simulink model "Template_v4_00_2023a_Jetson"  (R2023a)
settings: Solver=ode4  StartTime=0.0  StopTime=tsim  FixedStep=baseRate  RelTol=1e-6  AbsTol=1e-6
values from neighbouring files (symbols this model uses):
  a1 = shape(1)    [Cardioid.m]    (also in Run_Initializer.m = 0.3)
  a2 = shape(2)    [Cardioid.m]    (also in Run_Initializer.m = 0.3)
  a3 = shape(3)    [Cardioid.m]    (also in Run_Initializer.m = 0.4)
  b1 = shape(4)    [Cardioid.m]    (also in Run_Initializer.m = 0.175)
  b2 = shape(5)    [Cardioid.m]    (also in Run_Initializer.m = 0.175)
  drop_states_BLACK = BLACK_ini(1:3)    [Run_Initializer.m]
  drop_states_BLUE = BLUE_ini(1:3)    [Run_Initializer.m]
  drop_states_RED = RED_ini(1:3)    [Run_Initializer.m]
  Gamma1_el = 0.12    [Run_Initializer.m]
  Gamma1_sh = 0.005    [Run_Initializer.m]
  Gamma1_wr = 0.025    [Run_Initializer.m]
  Gamma2_el = 5    [Run_Initializer.m]
  Gamma2_sh = 5    [Run_Initializer.m]
  Gamma2_wr = 5    [Run_Initializer.m]
  Gamma3_el = 10    [Run_Initializer.m]
  Gamma3_sh = 40    [Run_Initializer.m]
  Gamma3_wr = 40    [Run_Initializer.m]
  Gamma4_el = 0.039    [Run_Initializer.m]
  Gamma4_sh = 0.015    [Run_Initializer.m]
  Gamma4_wr = 0.029    [Run_Initializer.m]
  Gamma5_el = 800    [Run_Initializer.m]
  Gamma5_sh = 800    [Run_Initializer.m]
  Gamma5_wr = 800    [Run_Initializer.m]
  Gamma6_el = 0.000001    (= 1e-06)    [Run_Initializer.m]
  Gamma6_sh = 0.005    [Run_Initializer.m]
  Gamma6_wr = 0.02    [Run_Initializer.m]
  home_states_BLACK = BLACK_ini(1:3)    [Run_Initializer.m]
  home_states_BLUE = BLUE_ini(1:3)    [Run_Initializer.m]
  home_states_RED = RED_ini(1:3)    [Run_Initializer.m]
  init_states_BLACK = BLACK_ini(1:3)    [Run_Initializer.m]
  init_states_BLUE = BLUE_ini(1:3)    [Run_Initializer.m]
  init_states_RED = RED_ini(1:3)    [Run_Initializer.m]
  Kd_elarm = 0.8    [Run_Initializer.m]
  Kd_sharm = 1.0    (= 1)    [Run_Initializer.m]
  Kd_wrarm = 0.6    [Run_Initializer.m]
  Kp_elarm = 1.2    [Run_Initializer.m]
  Kp_sharm = 1.5    [Run_Initializer.m]
  Kp_wrarm = 2    [Run_Initializer.m]
  PWMFreq = 5    [Run_Initializer.m]
  Tz_lim_elarm = .1    (= 0.1)    [Run_Initializer.m]
  Tz_lim_sharm = .1    (= 0.1)    [Run_Initializer.m]
  Tz_lim_wrarm = .1    (= 0.1)    [Run_Initializer.m]
undefined symbols (not defined in the file or in its folder): b0, b3, baseRate, DiscIntNeverNeededParam, drop_states_ARM, F_Black_X_nominal, F_Black_Y_nominal, F_Blue_X_nominal, F_Blue_Y_nominal, F_red_X_nominal, F_red_Y_nominal, F_thrusters_BLACK, F_thrusters_BLUE, F_thrusters_RED, IBLACK, IBLUE, IDIST, IEE, IPROX, IRED, Kd_tb, Kd_tblue, Kd_tr, Kd_xb, Kd_xblue, Kd_xr, Kd_yb, Kd_yblue, Kd_yr, Kp_tb, Kp_tblue, Kp_tr, Kp_xb, Kp_xblue, Kp_xr, Kp_yb, Kp_yblue, Kp_yr, mBLACK, mBLUE, mDIST, mEE, mPROX, mRED, noise_variance_BLACK, noise_variance_BLUE, noise_variance_RED, Phase0_End, Phase1_End, Phase2_End, Phase3_End, Phase3_SubPhase1_End, Phase3_SubPhase2_End, Phase3_SubPhase3_End, Phase3_SubPhase4_End, Phase4_End, Phase5_End, Phi, platformSelection, serverRate ... (+6)
libraries: nvidiaSharedBlocks x9, MainLibrary x4, dspsigops x4, simulink x1
(part 8 of 11)

== system Template_v4_00_2023a_Jetson/Phase #3: Experiment/Change BLACK Behavior/Sub-Phase #4/BLACK_RzD/Wrap1 ==
  unwrapped : Inport
  MATLAB Function : MATLAB Function  TreatAsAtomicUnit=on
  wrapped : Outport  VectorParamsAs1DForOutWhenUnconnected=off
  wires:
  MATLAB Function/1(wrappedAngle) -> wrapped/1
  unwrapped/1 -> MATLAB Function/1(u)

== system Template_v4_00_2023a_Jetson/Phase #3: Experiment/Change BLACK Behavior/Sub-Phase #4/Custom Discrete PD (Attitude)/x_dot -> x1 ==
  note: dy/dt ~= (y2-y1)/deltaT
  y(t) : Inport
  Delay1 : Delay  DelayLength=1  InitialConditionSource=Input port
      settings: InputPortMap=u0,p4
  Hold this value : Subsystem  TreatAsAtomicUnit=on
  Sum6 : Sum  Inputs=-+|
  divide by delta T : Gain  Gain=1/baseRate
  "if we went through a \"step\"" : If  IfExpression=u1 ~= 0  ShowElse=off
  dy(t)/dt : Outport  VectorParamsAs1DForOutWhenUnconnected=off
  wires:
  divide by delta T/1 -> dy(t)/dt/1
  Delay1/1 -> Sum6/1
  "if we went through a \"step\""/1 -> Hold this value/Action
  Hold this value/1(Out1) -> divide by delta T/1
  Sum6/1 -> "if we went through a \"step\""/1, Hold this value/1(In1)
  y(t)/1 -> Sum6/2, Delay1/2, Delay1/1

== system Template_v4_00_2023a_Jetson/Phase #3: Experiment/Change BLACK Behavior/Sub-Phase #4/Custom Discrete PD (X-Position)/x_dot -> x1 ==
  note: dy/dt ~= (y2-y1)/deltaT
  y(t) : Inport
  Delay1 : Delay  DelayLength=1  InitialConditionSource=Input port
      settings: InputPortMap=u0,p4
  Hold this value : Subsystem  TreatAsAtomicUnit=on
  Sum6 : Sum  Inputs=-+|
  divide by delta T : Gain  Gain=1/baseRate
  "if we went through a \"step\"" : If  IfExpression=u1 ~= 0  ShowElse=off
  dy(t)/dt : Outport  VectorParamsAs1DForOutWhenUnconnected=off
  wires:
  divide by delta T/1 -> dy(t)/dt/1
  Delay1/1 -> Sum6/1
  "if we went through a \"step\""/1 -> Hold this value/Action
  Hold this value/1(Out1) -> divide by delta T/1
  Sum6/1 -> "if we went through a \"step\""/1, Hold this value/1(In1)
  y(t)/1 -> Sum6/2, Delay1/2, Delay1/1

== system Template_v4_00_2023a_Jetson/Phase #3: Experiment/Change BLACK Behavior/Sub-Phase #4/Custom Discrete PD (Y-Position)/x_dot -> x1 ==
  note: dy/dt ~= (y2-y1)/deltaT
  y(t) : Inport
  Delay1 : Delay  DelayLength=1  InitialConditionSource=Input port
      settings: InputPortMap=u0,p4
  Hold this value : Subsystem  TreatAsAtomicUnit=on
  Sum6 : Sum  Inputs=-+|
  divide by delta T : Gain  Gain=1/baseRate
  "if we went through a \"step\"" : If  IfExpression=u1 ~= 0  ShowElse=off
  dy(t)/dt : Outport  VectorParamsAs1DForOutWhenUnconnected=off
  wires:
  divide by delta T/1 -> dy(t)/dt/1
  Delay1/1 -> Sum6/1
  "if we went through a \"step\""/1 -> Hold this value/Action
  Hold this value/1(Out1) -> divide by delta T/1
  Sum6/1 -> "if we went through a \"step\""/1, Hold this value/1(In1)
  y(t)/1 -> Sum6/2, Delay1/2, Delay1/1

== system Template_v4_00_2023a_Jetson/Phase #3: Experiment/Change BLUE Behavior/Sub-Phase #1/BLUE_Rz Desired/Subsystem ==
  Constant1 : Constant  Value=Phase2_End  SampleTime=-1
  Subtract : Sum  Inputs=+-
  Universal_Time : DataStoreRead  DataStoreName=Univ_Time  IndexOptions=Index vector (dialog)  Indices=1  OutputSizes=1
  Time : Outport  VectorParamsAs1DForOutWhenUnconnected=off
  wires:
  Universal_Time/1 -> Subtract/1
  Subtract/1 -> Time/1
  Constant1/1 -> Subtract/2

== system Template_v4_00_2023a_Jetson/Phase #3: Experiment/Change BLUE Behavior/Sub-Phase #1/BLUE_Rz Desired/Wrap ==
  unwrapped : Inport
  MATLAB Function : MATLAB Function  TreatAsAtomicUnit=on
  wrapped : Outport  VectorParamsAs1DForOutWhenUnconnected=off
  wires:
  MATLAB Function/1(wrappedAngle) -> wrapped/1
  unwrapped/1 -> MATLAB Function/1(u)

== system Template_v4_00_2023a_Jetson/Phase #3: Experiment/Change BLUE Behavior/Sub-Phase #1/Custom Discrete PD (Attitude)/x_dot -> x1 ==
  note: dy/dt ~= (y2-y1)/deltaT
  y(t) : Inport
  Delay1 : Delay  DelayLength=1  InitialConditionSource=Input port
      settings: InputPortMap=u0,p4
  Hold this value : Subsystem  TreatAsAtomicUnit=on
  Sum6 : Sum  Inputs=-+|
  divide by delta T : Gain  Gain=1/baseRate
  "if we went through a \"step\"" : If  IfExpression=u1 ~= 0  ShowElse=off
  dy(t)/dt : Outport  VectorParamsAs1DForOutWhenUnconnected=off
  wires:
  divide by delta T/1 -> dy(t)/dt/1
  Delay1/1 -> Sum6/1
  "if we went through a \"step\""/1 -> Hold this value/Action
  Hold this value/1(Out1) -> divide by delta T/1
  Sum6/1 -> "if we went through a \"step\""/1, Hold this value/1(In1)
  y(t)/1 -> Sum6/2, Delay1/2, Delay1/1

== system Template_v4_00_2023a_Jetson/Phase #3: Experiment/Change BLUE Behavior/Sub-Phase #1/Custom Discrete PD (X-Position)/x_dot -> x1 ==
  note: dy/dt ~= (y2-y1)/deltaT
  y(t) : Inport
  Delay1 : Delay  DelayLength=1  InitialConditionSource=Input port
      settings: InputPortMap=u0,p4
  Hold this value : Subsystem  TreatAsAtomicUnit=on
  Sum6 : Sum  Inputs=-+|
  divide by delta T : Gain  Gain=1/baseRate
  "if we went through a \"step\"" : If  IfExpression=u1 ~= 0  ShowElse=off
  dy(t)/dt : Outport  VectorParamsAs1DForOutWhenUnconnected=off
  wires:
  divide by delta T/1 -> dy(t)/dt/1
  Delay1/1 -> Sum6/1
  "if we went through a \"step\""/1 -> Hold this value/Action
  Hold this value/1(Out1) -> divide by delta T/1
  Sum6/1 -> "if we went through a \"step\""/1, Hold this value/1(In1)
  y(t)/1 -> Sum6/2, Delay1/2, Delay1/1

== system Template_v4_00_2023a_Jetson/Phase #3: Experiment/Change BLUE Behavior/Sub-Phase #1/Custom Discrete PD (Y-Position)/x_dot -> x1 ==
  note: dy/dt ~= (y2-y1)/deltaT
  y(t) : Inport
  Delay1 : Delay  DelayLength=1  InitialConditionSource=Input port
      settings: InputPortMap=u0,p4
  Hold this value : Subsystem  TreatAsAtomicUnit=on
  Sum6 : Sum  Inputs=-+|
  divide by delta T : Gain  Gain=1/baseRate
  "if we went through a \"step\"" : If  IfExpression=u1 ~= 0  ShowElse=off
  dy(t)/dt : Outport  VectorParamsAs1DForOutWhenUnconnected=off
  wires:
  divide by delta T/1 -> dy(t)/dt/1
  Delay1/1 -> Sum6/1
  "if we went through a \"step\""/1 -> Hold this value/Action
  Hold this value/1(Out1) -> divide by delta T/1
  Sum6/1 -> "if we went through a \"step\""/1, Hold this value/1(In1)
  y(t)/1 -> Sum6/2, Delay1/2, Delay1/1

== system Template_v4_00_2023a_Jetson/Phase #3: Experiment/Change BLUE Behavior/Sub-Phase #1/Subsystem2/Subsystem ==
  Universal_Time : DataStoreRead  DataStoreName=Univ_Time  IndexOptions=Index vector (dialog)  Indices=1  OutputSizes=1
  Time : Outport  VectorParamsAs1DForOutWhenUnconnected=off
  wires:
  Universal_Time/1 -> Time/1

== system Template_v4_00_2023a_Jetson/Phase #3: Experiment/Change BLUE Behavior/Sub-Phase #2 /BLUE_Rz Desired/Subsystem ==
  Constant1 : Constant  Value=Phase2_End  SampleTime=-1
  Subtract : Sum  Inputs=+-
  Universal_Time : DataStoreRead  DataStoreName=Univ_Time  IndexOptions=Index vector (dialog)  Indices=1  OutputSizes=1
  Time : Outport  VectorParamsAs1DForOutWhenUnconnected=off
  wires:
  Universal_Time/1 -> Subtract/1
  Subtract/1 -> Time/1
  Constant1/1 -> Subtract/2

== system Template_v4_00_2023a_Jetson/Phase #3: Experiment/Change BLUE Behavior/Sub-Phase #2 /BLUE_Rz Desired/Wrap ==
  unwrapped : Inport
  MATLAB Function : MATLAB Function  TreatAsAtomicUnit=on
  wrapped : Outport  VectorParamsAs1DForOutWhenUnconnected=off
  wires:
  MATLAB Function/1(wrappedAngle) -> wrapped/1
  unwrapped/1 -> MATLAB Function/1(u)

== system Template_v4_00_2023a_Jetson/Phase #3: Experiment/Change BLUE Behavior/Sub-Phase #2 /Custom Discrete PD (Attitude)/x_dot -> x1 ==
  note: dy/dt ~= (y2-y1)/deltaT
  y(t) : Inport
  Delay1 : Delay  DelayLength=1  InitialConditionSource=Input port
      settings: InputPortMap=u0,p4
  Hold this value : Subsystem  TreatAsAtomicUnit=on
  Sum6 : Sum  Inputs=-+|
  divide by delta T : Gain  Gain=1/baseRate
  "if we went through a \"step\"" : If  IfExpression=u1 ~= 0  ShowElse=off
  dy(t)/dt : Outport  VectorParamsAs1DForOutWhenUnconnected=off
  wires:
  divide by delta T/1 -> dy(t)/dt/1
  Delay1/1 -> Sum6/1
  "if we went through a \"step\""/1 -> Hold this value/Action
  Hold this value/1(Out1) -> divide by delta T/1
  Sum6/1 -> "if we went through a \"step\""/1, Hold this value/1(In1)
  y(t)/1 -> Sum6/2, Delay1/2, Delay1/1

== system Template_v4_00_2023a_Jetson/Phase #3: Experiment/Change BLUE Behavior/Sub-Phase #2 /Custom Discrete PD (X-Position)/x_dot -> x1 ==
  note: dy/dt ~= (y2-y1)/deltaT
  y(t) : Inport
  Delay1 : Delay  DelayLength=1  InitialConditionSource=Input port
      settings: InputPortMap=u0,p4
  Hold this value : Subsystem  TreatAsAtomicUnit=on
  Sum6 : Sum  Inputs=-+|
  divide by delta T : Gain  Gain=1/baseRate
  "if we went through a \"step\"" : If  IfExpression=u1 ~= 0  ShowElse=off
  dy(t)/dt : Outport  VectorParamsAs1DForOutWhenUnconnected=off
  wires:
  divide by delta T/1 -> dy(t)/dt/1
  Delay1/1 -> Sum6/1
  "if we went through a \"step\""/1 -> Hold this value/Action
  Hold this value/1(Out1) -> divide by delta T/1
  Sum6/1 -> "if we went through a \"step\""/1, Hold this value/1(In1)
  y(t)/1 -> Sum6/2, Delay1/2, Delay1/1

== system Template_v4_00_2023a_Jetson/Phase #3: Experiment/Change BLUE Behavior/Sub-Phase #2 /Custom Discrete PD (Y-Position)/x_dot -> x1 ==
  note: dy/dt ~= (y2-y1)/deltaT
  y(t) : Inport
  Delay1 : Delay  DelayLength=1  InitialConditionSource=Input port
      settings: InputPortMap=u0,p4
  Hold this value : Subsystem  TreatAsAtomicUnit=on
  Sum6 : Sum  Inputs=-+|
  divide by delta T : Gain  Gain=1/baseRate
  "if we went through a \"step\"" : If  IfExpression=u1 ~= 0  ShowElse=off
  dy(t)/dt : Outport  VectorParamsAs1DForOutWhenUnconnected=off
  wires:
  divide by delta T/1 -> dy(t)/dt/1
  Delay1/1 -> Sum6/1
  "if we went through a \"step\""/1 -> Hold this value/Action
  Hold this value/1(Out1) -> divide by delta T/1
  Sum6/1 -> "if we went through a \"step\""/1, Hold this value/1(In1)
  y(t)/1 -> Sum6/2, Delay1/2, Delay1/1

== system Template_v4_00_2023a_Jetson/Phase #3: Experiment/Change BLUE Behavior/Sub-Phase #2 /Subsystem2/Subsystem ==
  Universal_Time : DataStoreRead  DataStoreName=Univ_Time  IndexOptions=Index vector (dialog)  Indices=1  OutputSizes=1
  Time : Outport  VectorParamsAs1DForOutWhenUnconnected=off
  wires:
  Universal_Time/1 -> Time/1

== system Template_v4_00_2023a_Jetson/Phase #3: Experiment/Change BLUE Behavior/Sub-Phase #3 /BLUE_Rz Desired/Subsystem ==
  Constant1 : Constant  Value=Phase2_End  SampleTime=-1
  Subtract : Sum  Inputs=+-
  Universal_Time : DataStoreRead  DataStoreName=Univ_Time  IndexOptions=Index vector (dialog)  Indices=1  OutputSizes=1
  Time : Outport  VectorParamsAs1DForOutWhenUnconnected=off
  wires:
  Universal_Time/1 -> Subtract/1
  Subtract/1 -> Time/1
  Constant1/1 -> Subtract/2

== system Template_v4_00_2023a_Jetson/Phase #3: Experiment/Change BLUE Behavior/Sub-Phase #3 /BLUE_Rz Desired/Wrap ==
  unwrapped : Inport
  MATLAB Function : MATLAB Function  TreatAsAtomicUnit=on
  wrapped : Outport  VectorParamsAs1DForOutWhenUnconnected=off
  wires:
  MATLAB Function/1(wrappedAngle) -> wrapped/1
  unwrapped/1 -> MATLAB Function/1(u)

== system Template_v4_00_2023a_Jetson/Phase #3: Experiment/Change BLUE Behavior/Sub-Phase #3 /Custom Discrete PD (Attitude)/x_dot -> x1 ==
  note: dy/dt ~= (y2-y1)/deltaT
  y(t) : Inport
  Delay1 : Delay  DelayLength=1  InitialConditionSource=Input port
      settings: InputPortMap=u0,p4
  Hold this value : Subsystem  TreatAsAtomicUnit=on
  Sum6 : Sum  Inputs=-+|
  divide by delta T : Gain  Gain=1/baseRate
  "if we went through a \"step\"" : If  IfExpression=u1 ~= 0  ShowElse=off
  dy(t)/dt : Outport  VectorParamsAs1DForOutWhenUnconnected=off
  wires:
  divide by delta T/1 -> dy(t)/dt/1
  Delay1/1 -> Sum6/1
  "if we went through a \"step\""/1 -> Hold this value/Action
  Hold this value/1(Out1) -> divide by delta T/1
  Sum6/1 -> "if we went through a \"step\""/1, Hold this value/1(In1)
  y(t)/1 -> Sum6/2, Delay1/2, Delay1/1

== system Template_v4_00_2023a_Jetson/Phase #3: Experiment/Change BLUE Behavior/Sub-Phase #3 /Custom Discrete PD (X-Position)/x_dot -> x1 ==
  note: dy/dt ~= (y2-y1)/deltaT
  y(t) : Inport
  Delay1 : Delay  DelayLength=1  InitialConditionSource=Input port
      settings: InputPortMap=u0,p4
  Hold this value : Subsystem  TreatAsAtomicUnit=on
  Sum6 : Sum  Inputs=-+|
  divide by delta T : Gain  Gain=1/baseRate
  "if we went through a \"step\"" : If  IfExpression=u1 ~= 0  ShowElse=off
  dy(t)/dt : Outport  VectorParamsAs1DForOutWhenUnconnected=off
  wires:
  divide by delta T/1 -> dy(t)/dt/1
  Delay1/1 -> Sum6/1
  "if we went through a \"step\""/1 -> Hold this value/Action
  Hold this value/1(Out1) -> divide by delta T/1
  Sum6/1 -> "if we went through a \"step\""/1, Hold this value/1(In1)
  y(t)/1 -> Sum6/2, Delay1/2, Delay1/1

== system Template_v4_00_2023a_Jetson/Phase #3: Experiment/Change BLUE Behavior/Sub-Phase #3 /Custom Discrete PD (Y-Position)/x_dot -> x1 ==
  note: dy/dt ~= (y2-y1)/deltaT
  y(t) : Inport
  Delay1 : Delay  DelayLength=1  InitialConditionSource=Input port
      settings: InputPortMap=u0,p4
  Hold this value : Subsystem  TreatAsAtomicUnit=on
  Sum6 : Sum  Inputs=-+|
  divide by delta T : Gain  Gain=1/baseRate
  "if we went through a \"step\"" : If  IfExpression=u1 ~= 0  ShowElse=off
  dy(t)/dt : Outport  VectorParamsAs1DForOutWhenUnconnected=off
  wires:
  divide by delta T/1 -> dy(t)/dt/1
  Delay1/1 -> Sum6/1
  "if we went through a \"step\""/1 -> Hold this value/Action
  Hold this value/1(Out1) -> divide by delta T/1
  Sum6/1 -> "if we went through a \"step\""/1, Hold this value/1(In1)
  y(t)/1 -> Sum6/2, Delay1/2, Delay1/1

== system Template_v4_00_2023a_Jetson/Phase #3: Experiment/Change BLUE Behavior/Sub-Phase #3 /Subsystem2/Subsystem ==
  Universal_Time : DataStoreRead  DataStoreName=Univ_Time  IndexOptions=Index vector (dialog)  Indices=1  OutputSizes=1
  Time : Outport  VectorParamsAs1DForOutWhenUnconnected=off
  wires:
  Universal_Time/1 -> Time/1

== system Template_v4_00_2023a_Jetson/Phase #3: Experiment/Change BLUE Behavior/Sub-Phase #4/BLUE_Rz Desired/Subsystem ==
  Constant1 : Constant  Value=Phase2_End  SampleTime=-1
  Subtract : Sum  Inputs=+-
  Universal_Time : DataStoreRead  DataStoreName=Univ_Time  IndexOptions=Index vector (dialog)  Indices=1  OutputSizes=1
  Time : Outport  VectorParamsAs1DForOutWhenUnconnected=off
  wires:
  Universal_Time/1 -> Subtract/1
  Subtract/1 -> Time/1
  Constant1/1 -> Subtract/2

== system Template_v4_00_2023a_Jetson/Phase #3: Experiment/Change BLUE Behavior/Sub-Phase #4/BLUE_Rz Desired/Wrap ==
  unwrapped : Inport
  MATLAB Function : MATLAB Function  TreatAsAtomicUnit=on
  wrapped : Outport  VectorParamsAs1DForOutWhenUnconnected=off
  wires:
  MATLAB Function/1(wrappedAngle) -> wrapped/1
  unwrapped/1 -> MATLAB Function/1(u)

== system Template_v4_00_2023a_Jetson/Phase #3: Experiment/Change BLUE Behavior/Sub-Phase #4/Custom Discrete PD (Attitude)/x_dot -> x1 ==
  note: dy/dt ~= (y2-y1)/deltaT
  y(t) : Inport
  Delay1 : Delay  DelayLength=1  InitialConditionSource=Input port
      settings: InputPortMap=u0,p4
  Hold this value : Subsystem  TreatAsAtomicUnit=on
  Sum6 : Sum  Inputs=-+|
  divide by delta T : Gain  Gain=1/baseRate
  "if we went through a \"step\"" : If  IfExpression=u1 ~= 0  ShowElse=off
  dy(t)/dt : Outport  VectorParamsAs1DForOutWhenUnconnected=off
  wires:
  divide by delta T/1 -> dy(t)/dt/1
  Delay1/1 -> Sum6/1
  "if we went through a \"step\""/1 -> Hold this value/Action
  Hold this value/1(Out1) -> divide by delta T/1
  Sum6/1 -> "if we went through a \"step\""/1, Hold this value/1(In1)
  y(t)/1 -> Sum6/2, Delay1/2, Delay1/1

== system Template_v4_00_2023a_Jetson/Phase #3: Experiment/Change BLUE Behavior/Sub-Phase #4/Custom Discrete PD (X-Position)/x_dot -> x1 ==
  note: dy/dt ~= (y2-y1)/deltaT
  y(t) : Inport
  Delay1 : Delay  DelayLength=1  InitialConditionSource=Input port
      settings: InputPortMap=u0,p4
  Hold this value : Subsystem  TreatAsAtomicUnit=on
  Sum6 : Sum  Inputs=-+|
  divide by delta T : Gain  Gain=1/baseRate
  "if we went through a \"step\"" : If  IfExpression=u1 ~= 0  ShowElse=off
  dy(t)/dt : Outport  VectorParamsAs1DForOutWhenUnconnected=off
  wires:
  divide by delta T/1 -> dy(t)/dt/1
  Delay1/1 -> Sum6/1
  "if we went through a \"step\""/1 -> Hold this value/Action
  Hold this value/1(Out1) -> divide by delta T/1
  Sum6/1 -> "if we went through a \"step\""/1, Hold this value/1(In1)
  y(t)/1 -> Sum6/2, Delay1/2, Delay1/1

== system Template_v4_00_2023a_Jetson/Phase #3: Experiment/Change BLUE Behavior/Sub-Phase #4/Custom Discrete PD (Y-Position)/x_dot -> x1 ==
  note: dy/dt ~= (y2-y1)/deltaT
  y(t) : Inport
  Delay1 : Delay  DelayLength=1  InitialConditionSource=Input port
      settings: InputPortMap=u0,p4
  Hold this value : Subsystem  TreatAsAtomicUnit=on
  Sum6 : Sum  Inputs=-+|
  divide by delta T : Gain  Gain=1/baseRate
  "if we went through a \"step\"" : If  IfExpression=u1 ~= 0  ShowElse=off
  dy(t)/dt : Outport  VectorParamsAs1DForOutWhenUnconnected=off
  wires:
  divide by delta T/1 -> dy(t)/dt/1
  Delay1/1 -> Sum6/1
  "if we went through a \"step\""/1 -> Hold this value/Action
  Hold this value/1(Out1) -> divide by delta T/1
  Sum6/1 -> "if we went through a \"step\""/1, Hold this value/1(In1)
  y(t)/1 -> Sum6/2, Delay1/2, Delay1/1

== system Template_v4_00_2023a_Jetson/Phase #3: Experiment/Change BLUE Behavior/Sub-Phase #4/Subsystem2/Subsystem ==
  Universal_Time : DataStoreRead  DataStoreName=Univ_Time  IndexOptions=Index vector (dialog)  Indices=1  OutputSizes=1
  Time : Outport  VectorParamsAs1DForOutWhenUnconnected=off
  wires:
  Universal_Time/1 -> Time/1

== system Template_v4_00_2023a_Jetson/Phase #3: Experiment/Change RED Behavior/Sub-Phase #1/Custom Discrete PD (Attitude)/x_dot -> x2 ==
  note: dy/dt ~= (y2-y1)/deltaT
  y(t) : Inport
  Delay1 : Delay  DelayLength=1  InitialConditionSource=Input port
      settings: InputPortMap=u0,p4
  Hold this value : Subsystem  TreatAsAtomicUnit=on
  Sum6 : Sum  Inputs=-+|
  divide by delta T : Gain  Gain=1/baseRate
  "if we went through a \"step\"" : If  IfExpression=u1 ~= 0  ShowElse=off
  dy(t)/dt : Outport  VectorParamsAs1DForOutWhenUnconnected=off
  wires:
  divide by delta T/1 -> dy(t)/dt/1
  Delay1/1 -> Sum6/1
  "if we went through a \"step\""/1 -> Hold this value/Action
  Hold this value/1(Out1) -> divide by delta T/1
  Sum6/1 -> "if we went through a \"step\""/1, Hold this value/1(In1)
  y(t)/1 -> Sum6/2, Delay1/2, Delay1/1

== system Template_v4_00_2023a_Jetson/Phase #3: Experiment/Change RED Behavior/Sub-Phase #1/Custom Discrete PD (X-Position)/x_dot -> x2 ==
  note: dy/dt ~= (y2-y1)/deltaT
  y(t) : Inport
  Delay1 : Delay  DelayLength=1  InitialConditionSource=Input port
      settings: InputPortMap=u0,p4
  Hold this value : Subsystem  TreatAsAtomicUnit=on
  Sum6 : Sum  Inputs=-+|
  divide by delta T : Gain  Gain=1/baseRate
  "if we went through a \"step\"" : If  IfExpression=u1 ~= 0  ShowElse=off
  dy(t)/dt : Outport  VectorParamsAs1DForOutWhenUnconnected=off
  wires:
  divide by delta T/1 -> dy(t)/dt/1
  Delay1/1 -> Sum6/1
  "if we went through a \"step\""/1 -> Hold this value/Action
  Hold this value/1(Out1) -> divide by delta T/1
  Sum6/1 -> "if we went through a \"step\""/1, Hold this value/1(In1)
  y(t)/1 -> Sum6/2, Delay1/2, Delay1/1

== system Template_v4_00_2023a_Jetson/Phase #3: Experiment/Change RED Behavior/Sub-Phase #1/Custom Discrete PD (Y-Position)/x_dot -> x2 ==
  note: dy/dt ~= (y2-y1)/deltaT
  y(t) : Inport
  Delay1 : Delay  DelayLength=1  InitialConditionSource=Input port
      settings: InputPortMap=u0,p4
  Hold this value : Subsystem  TreatAsAtomicUnit=on
  Sum6 : Sum  Inputs=-+|
  divide by delta T : Gain  Gain=1/baseRate
  "if we went through a \"step\"" : If  IfExpression=u1 ~= 0  ShowElse=off
  dy(t)/dt : Outport  VectorParamsAs1DForOutWhenUnconnected=off
  wires:
  divide by delta T/1 -> dy(t)/dt/1
  Delay1/1 -> Sum6/1
  "if we went through a \"step\""/1 -> Hold this value/Action
  Hold this value/1(Out1) -> divide by delta T/1
  Sum6/1 -> "if we went through a \"step\""/1, Hold this value/1(In1)
  y(t)/1 -> Sum6/2, Delay1/2, Delay1/1

== system Template_v4_00_2023a_Jetson/Phase #3: Experiment/Change RED Behavior/Sub-Phase #1/RED+ARM/Passthrough for Experiment ==
  q1_desired : Inport
  q2_desired : Inport  Port=2
  q3_desired : Inport  Port=3
  Action Port : ActionPort  ActionPortLabel=else
  q1_command : Outport
  q2_command : Outport  Port=2
  q3_command : Outport  Port=3
  wires:
  q3_desired/1 -> q3_command/1
  q1_desired/1 -> q1_command/1
  q2_desired/1 -> q2_command/1

== system Template_v4_00_2023a_Jetson/Phase #3: Experiment/Change RED Behavior/Sub-Phase #1/RED+ARM/Simulated Position Controller ==
  q1_desired : Inport
  q2_desired : Inport  Port=2
  q3_desired : Inport  Port=3
  Action Port : ActionPort  ActionPortLabel=if(u1 == 1)
  Custom Discrete PD (Elbow) : Subsystem
  Custom Discrete PD (Shoulder) : Subsystem
  Custom Discrete PD (Wrist) : Subsystem
  Data Store Read : DataStoreRead  DataStoreName=RED_Rz_Shoulder  IndexOptions=Index vector (dialog)  Indices=1  OutputSizes=1
  Data Store Read5 : DataStoreRead  DataStoreName=RED_Rz_Elbow  IndexOptions=Index vector (dialog)  Indices=1  OutputSizes=1
  Data Store Read6 : DataStoreRead  DataStoreName=RED_Rz_Wrist  IndexOptions=Index vector (dialog)  Indices=1  OutputSizes=1
  Saturation : Saturate  UpperLimit=Tz_lim_sharm  LowerLimit=-Tz_lim_sharm
  Saturation1 : Saturate  UpperLimit=Tz_lim_elarm  LowerLimit=-Tz_lim_elarm
  Saturation3 : Saturate  UpperLimit=Tz_lim_wrarm  LowerLimit=-Tz_lim_wrarm
  Subtract2 : Sum  Inputs=+-
  Subtract3 : Sum  Inputs=+-
  Subtract4 : Sum  Inputs=+-
  q1_command : Outport
  q2_command : Outport  Port=2
  q3_command : Outport  Port=3
  wires:
  Saturation3/1 -> q3_command/1
  Subtract4/1 -> Custom Discrete PD (Wrist)/1(ey)
  Custom Discrete PD (Shoulder)/1(Fx) -> Saturation/1
  Custom Discrete PD (Elbow)/1(Fy) -> Saturation1/1
  Saturation/1 -> q1_command/1
  Subtract2/1 -> Custom Discrete PD (Shoulder)/1(ex)
  Saturation1/1 -> q2_command/1
  Custom Discrete PD (Wrist)/1(Fy) -> Saturation3/1
  Subtract3/1 -> Custom Discrete PD (Elbow)/1(ey)
  Data Store Read/1 -> Subtract2/2
  Data Store Read5/1 -> Subtract3/2
  Data Store Read6/1 -> Subtract4/2
  q1_desired/1 -> Subtract2/1
  q2_desired/1 -> Subtract3/1
  q3_desired/1 -> Subtract4/1

== system Template_v4_00_2023a_Jetson/Phase #3: Experiment/Change RED Behavior/Sub-Phase #1/RED_Rz Desired/Subsystem ==
  Constant1 : Constant  Value=Phase2_End  SampleTime=-1
  Subtract : Sum  Inputs=+-
  Universal_Time : DataStoreRead  DataStoreName=Univ_Time  IndexOptions=Index vector (dialog)  Indices=1  OutputSizes=1
  Time : Outport  VectorParamsAs1DForOutWhenUnconnected=off
  wires:
  Universal_Time/1 -> Subtract/1
  Subtract/1 -> Time/1
  Constant1/1 -> Subtract/2

== system Template_v4_00_2023a_Jetson/Phase #3: Experiment/Change RED Behavior/Sub-Phase #1/RED_Rz Desired/Wrap ==
  unwrapped : Inport
  MATLAB Function : MATLAB Function  TreatAsAtomicUnit=on
  wrapped : Outport  VectorParamsAs1DForOutWhenUnconnected=off
  wires:
  MATLAB Function/1(wrappedAngle) -> wrapped/1
  unwrapped/1 -> MATLAB Function/1(u)

== system Template_v4_00_2023a_Jetson/Phase #3: Experiment/Change RED Behavior/Sub-Phase #1/Subsystem1/Subsystem ==
  Universal_Time : DataStoreRead  DataStoreName=Univ_Time  IndexOptions=Index vector (dialog)  Indices=1  OutputSizes=1
  Time : Outport  VectorParamsAs1DForOutWhenUnconnected=off
  wires:
  Universal_Time/1 -> Time/1

== system Template_v4_00_2023a_Jetson/Phase #3: Experiment/Change RED Behavior/Sub-Phase #2 /Custom Discrete PD (Attitude)/x_dot -> x2 ==
  note: dy/dt ~= (y2-y1)/deltaT
  y(t) : Inport
  Delay1 : Delay  DelayLength=1  InitialConditionSource=Input port
      settings: InputPortMap=u0,p4
  Hold this value : Subsystem  TreatAsAtomicUnit=on
  Sum6 : Sum  Inputs=-+|
  divide by delta T : Gain  Gain=1/baseRate
  "if we went through a \"step\"" : If  IfExpression=u1 ~= 0  ShowElse=off
  dy(t)/dt : Outport  VectorParamsAs1DForOutWhenUnconnected=off
  wires:
  divide by delta T/1 -> dy(t)/dt/1
  Delay1/1 -> Sum6/1
  "if we went through a \"step\""/1 -> Hold this value/Action
  Hold this value/1(Out1) -> divide by delta T/1
  Sum6/1 -> "if we went through a \"step\""/1, Hold this value/1(In1)
  y(t)/1 -> Sum6/2, Delay1/2, Delay1/1

== system Template_v4_00_2023a_Jetson/Phase #3: Experiment/Change RED Behavior/Sub-Phase #2 /Custom Discrete PD (X-Position)/x_dot -> x2 ==
  note: dy/dt ~= (y2-y1)/deltaT
  y(t) : Inport
  Delay1 : Delay  DelayLength=1  InitialConditionSource=Input port
      settings: InputPortMap=u0,p4
  Hold this value : Subsystem  TreatAsAtomicUnit=on
  Sum6 : Sum  Inputs=-+|
  divide by delta T : Gain  Gain=1/baseRate
  "if we went through a \"step\"" : If  IfExpression=u1 ~= 0  ShowElse=off
  dy(t)/dt : Outport  VectorParamsAs1DForOutWhenUnconnected=off
  wires:
  divide by delta T/1 -> dy(t)/dt/1
  Delay1/1 -> Sum6/1
  "if we went through a \"step\""/1 -> Hold this value/Action
  Hold this value/1(Out1) -> divide by delta T/1
  Sum6/1 -> "if we went through a \"step\""/1, Hold this value/1(In1)
  y(t)/1 -> Sum6/2, Delay1/2, Delay1/1

== system Template_v4_00_2023a_Jetson/Phase #3: Experiment/Change RED Behavior/Sub-Phase #2 /Custom Discrete PD (Y-Position)/x_dot -> x2 ==
  note: dy/dt ~= (y2-y1)/deltaT
  y(t) : Inport
  Delay1 : Delay  DelayLength=1  InitialConditionSource=Input port
      settings: InputPortMap=u0,p4
  Hold this value : Subsystem  TreatAsAtomicUnit=on
  Sum6 : Sum  Inputs=-+|
  divide by delta T : Gain  Gain=1/baseRate
  "if we went through a \"step\"" : If  IfExpression=u1 ~= 0  ShowElse=off
  dy(t)/dt : Outport  VectorParamsAs1DForOutWhenUnconnected=off
  wires:
  divide by delta T/1 -> dy(t)/dt/1
  Delay1/1 -> Sum6/1
  "if we went through a \"step\""/1 -> Hold this value/Action
  Hold this value/1(Out1) -> divide by delta T/1
  Sum6/1 -> "if we went through a \"step\""/1, Hold this value/1(In1)
  y(t)/1 -> Sum6/2, Delay1/2, Delay1/1

== system Template_v4_00_2023a_Jetson/Phase #3: Experiment/Change RED Behavior/Sub-Phase #2 /RED+ARM/Passthrough for Experiment ==
  q1_desired : Inport
  q2_desired : Inport  Port=2
  q3_desired : Inport  Port=3
  Action Port : ActionPort  ActionPortLabel=else
  q1_command : Outport
  q2_command : Outport  Port=2
  q3_command : Outport  Port=3
  wires:
  q3_desired/1 -> q3_command/1
  q1_desired/1 -> q1_command/1
  q2_desired/1 -> q2_command/1

== system Template_v4_00_2023a_Jetson/Phase #3: Experiment/Change RED Behavior/Sub-Phase #2 /RED+ARM/Simulated Position Controller ==
  q1_desired : Inport
  q2_desired : Inport  Port=2
  q3_desired : Inport  Port=3
  Action Port : ActionPort  ActionPortLabel=if(u1 == 1)
  Custom Discrete PD (Elbow) : Subsystem
  Custom Discrete PD (Shoulder) : Subsystem
  Custom Discrete PD (Wrist) : Subsystem
  Data Store Read : DataStoreRead  DataStoreName=RED_Rz_Shoulder  IndexOptions=Index vector (dialog)  Indices=1  OutputSizes=1
  Data Store Read5 : DataStoreRead  DataStoreName=RED_Rz_Elbow  IndexOptions=Index vector (dialog)  Indices=1  OutputSizes=1
  Data Store Read6 : DataStoreRead  DataStoreName=RED_Rz_Wrist  IndexOptions=Index vector (dialog)  Indices=1  OutputSizes=1
  Saturation : Saturate  UpperLimit=Tz_lim_sharm  LowerLimit=-Tz_lim_sharm
  Saturation1 : Saturate  UpperLimit=Tz_lim_elarm  LowerLimit=-Tz_lim_elarm
  Saturation3 : Saturate  UpperLimit=Tz_lim_wrarm  LowerLimit=-Tz_lim_wrarm
  Subtract2 : Sum  Inputs=+-
  Subtract3 : Sum  Inputs=+-
  Subtract4 : Sum  Inputs=+-
  q1_command : Outport
  q2_command : Outport  Port=2
  q3_command : Outport  Port=3
  wires:
  Saturation3/1 -> q3_command/1
  Subtract4/1 -> Custom Discrete PD (Wrist)/1(ey)
  Custom Discrete PD (Shoulder)/1(Fx) -> Saturation/1
  Custom Discrete PD (Elbow)/1(Fy) -> Saturation1/1
  Saturation/1 -> q1_command/1
  Subtract2/1 -> Custom Discrete PD (Shoulder)/1(ex)
  Saturation1/1 -> q2_command/1
  Custom Discrete PD (Wrist)/1(Fy) -> Saturation3/1
  Subtract3/1 -> Custom Discrete PD (Elbow)/1(ey)
  Data Store Read/1 -> Subtract2/2
  Data Store Read5/1 -> Subtract3/2
  Data Store Read6/1 -> Subtract4/2
  q1_desired/1 -> Subtract2/1
  q2_desired/1 -> Subtract3/1
  q3_desired/1 -> Subtract4/1

== system Template_v4_00_2023a_Jetson/Phase #3: Experiment/Change RED Behavior/Sub-Phase #2 /RED_Rz Desired/Subsystem ==
  Constant1 : Constant  Value=Phase2_End  SampleTime=-1
  Subtract : Sum  Inputs=+-
  Universal_Time : DataStoreRead  DataStoreName=Univ_Time  IndexOptions=Index vector (dialog)  Indices=1  OutputSizes=1
  Time : Outport  VectorParamsAs1DForOutWhenUnconnected=off
  wires:
  Universal_Time/1 -> Subtract/1
  Subtract/1 -> Time/1
  Constant1/1 -> Subtract/2

== system Template_v4_00_2023a_Jetson/Phase #3: Experiment/Change RED Behavior/Sub-Phase #2 /RED_Rz Desired/Wrap ==
  unwrapped : Inport
  MATLAB Function : MATLAB Function  TreatAsAtomicUnit=on
  wrapped : Outport  VectorParamsAs1DForOutWhenUnconnected=off
  wires:
  MATLAB Function/1(wrappedAngle) -> wrapped/1
  unwrapped/1 -> MATLAB Function/1(u)

== system Template_v4_00_2023a_Jetson/Phase #3: Experiment/Change RED Behavior/Sub-Phase #2 /Subsystem1/Subsystem ==
  Universal_Time : DataStoreRead  DataStoreName=Univ_Time  IndexOptions=Index vector (dialog)  Indices=1  OutputSizes=1
  Time : Outport  VectorParamsAs1DForOutWhenUnconnected=off
  wires:
  Universal_Time/1 -> Time/1

== system Template_v4_00_2023a_Jetson/Phase #3: Experiment/Change RED Behavior/Sub-Phase #3 /Custom Discrete PD (Attitude)/x_dot -> x2 ==
  note: dy/dt ~= (y2-y1)/deltaT
  y(t) : Inport
  Delay1 : Delay  DelayLength=1  InitialConditionSource=Input port
      settings: InputPortMap=u0,p4
  Hold this value : Subsystem  TreatAsAtomicUnit=on
  Sum6 : Sum  Inputs=-+|
  divide by delta T : Gain  Gain=1/baseRate
  "if we went through a \"step\"" : If  IfExpression=u1 ~= 0  ShowElse=off
  dy(t)/dt : Outport  VectorParamsAs1DForOutWhenUnconnected=off
  wires:
  divide by delta T/1 -> dy(t)/dt/1
  Delay1/1 -> Sum6/1
  "if we went through a \"step\""/1 -> Hold this value/Action
  Hold this value/1(Out1) -> divide by delta T/1
  Sum6/1 -> "if we went through a \"step\""/1, Hold this value/1(In1)
  y(t)/1 -> Sum6/2, Delay1/2, Delay1/1

== system Template_v4_00_2023a_Jetson/Phase #3: Experiment/Change RED Behavior/Sub-Phase #3 /Custom Discrete PD (X-Position)/x_dot -> x2 ==
  note: dy/dt ~= (y2-y1)/deltaT
  y(t) : Inport
  Delay1 : Delay  DelayLength=1  InitialConditionSource=Input port
      settings: InputPortMap=u0,p4
  Hold this value : Subsystem  TreatAsAtomicUnit=on
  Sum6 : Sum  Inputs=-+|
  divide by delta T : Gain  Gain=1/baseRate
  "if we went through a \"step\"" : If  IfExpression=u1 ~= 0  ShowElse=off
  dy(t)/dt : Outport  VectorParamsAs1DForOutWhenUnconnected=off
  wires:
  divide by delta T/1 -> dy(t)/dt/1
  Delay1/1 -> Sum6/1
  "if we went through a \"step\""/1 -> Hold this value/Action
  Hold this value/1(Out1) -> divide by delta T/1
  Sum6/1 -> "if we went through a \"step\""/1, Hold this value/1(In1)
  y(t)/1 -> Sum6/2, Delay1/2, Delay1/1

== system Template_v4_00_2023a_Jetson/Phase #3: Experiment/Change RED Behavior/Sub-Phase #3 /Custom Discrete PD (Y-Position)/x_dot -> x2 ==
  note: dy/dt ~= (y2-y1)/deltaT
  y(t) : Inport
  Delay1 : Delay  DelayLength=1  InitialConditionSource=Input port
      settings: InputPortMap=u0,p4
  Hold this value : Subsystem  TreatAsAtomicUnit=on
  Sum6 : Sum  Inputs=-+|
  divide by delta T : Gain  Gain=1/baseRate
  "if we went through a \"step\"" : If  IfExpression=u1 ~= 0  ShowElse=off
  dy(t)/dt : Outport  VectorParamsAs1DForOutWhenUnconnected=off
  wires:
  divide by delta T/1 -> dy(t)/dt/1
  Delay1/1 -> Sum6/1
  "if we went through a \"step\""/1 -> Hold this value/Action
  Hold this value/1(Out1) -> divide by delta T/1
  Sum6/1 -> "if we went through a \"step\""/1, Hold this value/1(In1)
  y(t)/1 -> Sum6/2, Delay1/2, Delay1/1

== system Template_v4_00_2023a_Jetson/Phase #3: Experiment/Change RED Behavior/Sub-Phase #3 /RED+ARM/Passthrough for Experiment ==
  q1_desired : Inport
  q2_desired : Inport  Port=2
  q3_desired : Inport  Port=3
  Action Port : ActionPort  ActionPortLabel=else
  q1_command : Outport
  q2_command : Outport  Port=2
  q3_command : Outport  Port=3
  wires:
  q3_desired/1 -> q3_command/1
  q1_desired/1 -> q1_command/1
  q2_desired/1 -> q2_command/1

== system Template_v4_00_2023a_Jetson/Phase #3: Experiment/Change RED Behavior/Sub-Phase #3 /RED+ARM/Simulated Position Controller ==
  q1_desired : Inport
  q2_desired : Inport  Port=2
  q3_desired : Inport  Port=3
  Action Port : ActionPort  ActionPortLabel=if(u1 == 1)
  Custom Discrete PD (Elbow) : Subsystem
  Custom Discrete PD (Shoulder) : Subsystem
  Custom Discrete PD (Wrist) : Subsystem
  Data Store Read : DataStoreRead  DataStoreName=RED_Rz_Shoulder  IndexOptions=Index vector (dialog)  Indices=1  OutputSizes=1
  Data Store Read5 : DataStoreRead  DataStoreName=RED_Rz_Elbow  IndexOptions=Index vector (dialog)  Indices=1  OutputSizes=1
  Data Store Read6 : DataStoreRead  DataStoreName=RED_Rz_Wrist  IndexOptions=Index vector (dialog)  Indices=1  OutputSizes=1
  Saturation : Saturate  UpperLimit=Tz_lim_sharm  LowerLimit=-Tz_lim_sharm
  Saturation1 : Saturate  UpperLimit=Tz_lim_elarm  LowerLimit=-Tz_lim_elarm
  Saturation3 : Saturate  UpperLimit=Tz_lim_wrarm  LowerLimit=-Tz_lim_wrarm
  Subtract2 : Sum  Inputs=+-
  Subtract3 : Sum  Inputs=+-
  Subtract4 : Sum  Inputs=+-
  q1_command : Outport
  q2_command : Outport  Port=2
  q3_command : Outport  Port=3
  wires:
  Saturation3/1 -> q3_command/1
  Subtract4/1 -> Custom Discrete PD (Wrist)/1(ey)
  Custom Discrete PD (Shoulder)/1(Fx) -> Saturation/1
  Custom Discrete PD (Elbow)/1(Fy) -> Saturation1/1
  Saturation/1 -> q1_command/1
  Subtract2/1 -> Custom Discrete PD (Shoulder)/1(ex)
  Saturation1/1 -> q2_command/1
  Custom Discrete PD (Wrist)/1(Fy) -> Saturation3/1
  Subtract3/1 -> Custom Discrete PD (Elbow)/1(ey)
  Data Store Read/1 -> Subtract2/2
  Data Store Read5/1 -> Subtract3/2
  Data Store Read6/1 -> Subtract4/2
  q1_desired/1 -> Subtract2/1
  q2_desired/1 -> Subtract3/1
  q3_desired/1 -> Subtract4/1

== system Template_v4_00_2023a_Jetson/Phase #3: Experiment/Change RED Behavior/Sub-Phase #3 /RED_Rz Desired/Subsystem ==
  Constant1 : Constant  Value=Phase2_End  SampleTime=-1
  Subtract : Sum  Inputs=+-
  Universal_Time : DataStoreRead  DataStoreName=Univ_Time  IndexOptions=Index vector (dialog)  Indices=1  OutputSizes=1
  Time : Outport  VectorParamsAs1DForOutWhenUnconnected=off
  wires:
  Universal_Time/1 -> Subtract/1
  Subtract/1 -> Time/1
  Constant1/1 -> Subtract/2

== system Template_v4_00_2023a_Jetson/Phase #3: Experiment/Change RED Behavior/Sub-Phase #3 /RED_Rz Desired/Wrap ==
  unwrapped : Inport
  MATLAB Function : MATLAB Function  TreatAsAtomicUnit=on
  wrapped : Outport  VectorParamsAs1DForOutWhenUnconnected=off
  wires:
  MATLAB Function/1(wrappedAngle) -> wrapped/1
  unwrapped/1 -> MATLAB Function/1(u)

== system Template_v4_00_2023a_Jetson/Phase #3: Experiment/Change RED Behavior/Sub-Phase #3 /Subsystem1/Subsystem ==
  Universal_Time : DataStoreRead  DataStoreName=Univ_Time  IndexOptions=Index vector (dialog)  Indices=1  OutputSizes=1
  Time : Outport  VectorParamsAs1DForOutWhenUnconnected=off
  wires:
  Universal_Time/1 -> Time/1

== system Template_v4_00_2023a_Jetson/Phase #3: Experiment/Change RED Behavior/Sub-Phase #4/Custom Discrete PD (Attitude)/x_dot -> x2 ==
  note: dy/dt ~= (y2-y1)/deltaT
  y(t) : Inport
  Delay1 : Delay  DelayLength=1  InitialConditionSource=Input port
      settings: InputPortMap=u0,p4
  Hold this value : Subsystem  TreatAsAtomicUnit=on
  Sum6 : Sum  Inputs=-+|
  divide by delta T : Gain  Gain=1/baseRate
  "if we went through a \"step\"" : If  IfExpression=u1 ~= 0  ShowElse=off
  dy(t)/dt : Outport  VectorParamsAs1DForOutWhenUnconnected=off
  wires:
  divide by delta T/1 -> dy(t)/dt/1
  Delay1/1 -> Sum6/1
  "if we went through a \"step\""/1 -> Hold this value/Action
  Hold this value/1(Out1) -> divide by delta T/1
  Sum6/1 -> "if we went through a \"step\""/1, Hold this value/1(In1)
  y(t)/1 -> Sum6/2, Delay1/2, Delay1/1

== system Template_v4_00_2023a_Jetson/Phase #3: Experiment/Change RED Behavior/Sub-Phase #4/Custom Discrete PD (X-Position)/x_dot -> x2 ==
  note: dy/dt ~= (y2-y1)/deltaT
  y(t) : Inport
  Delay1 : Delay  DelayLength=1  InitialConditionSource=Input port
      settings: InputPortMap=u0,p4
  Hold this value : Subsystem  TreatAsAtomicUnit=on
  Sum6 : Sum  Inputs=-+|
  divide by delta T : Gain  Gain=1/baseRate
  "if we went through a \"step\"" : If  IfExpression=u1 ~= 0  ShowElse=off
  dy(t)/dt : Outport  VectorParamsAs1DForOutWhenUnconnected=off
  wires:
  divide by delta T/1 -> dy(t)/dt/1
  Delay1/1 -> Sum6/1
  "if we went through a \"step\""/1 -> Hold this value/Action
  Hold this value/1(Out1) -> divide by delta T/1
  Sum6/1 -> "if we went through a \"step\""/1, Hold this value/1(In1)
  y(t)/1 -> Sum6/2, Delay1/2, Delay1/1

== system Template_v4_00_2023a_Jetson/Phase #3: Experiment/Change RED Behavior/Sub-Phase #4/Custom Discrete PD (Y-Position)/x_dot -> x2 ==
  note: dy/dt ~= (y2-y1)/deltaT
  y(t) : Inport
  Delay1 : Delay  DelayLength=1  InitialConditionSource=Input port
      settings: InputPortMap=u0,p4
  Hold this value : Subsystem  TreatAsAtomicUnit=on
  Sum6 : Sum  Inputs=-+|
  divide by delta T : Gain  Gain=1/baseRate
  "if we went through a \"step\"" : If  IfExpression=u1 ~= 0  ShowElse=off
  dy(t)/dt : Outport  VectorParamsAs1DForOutWhenUnconnected=off
  wires:
  divide by delta T/1 -> dy(t)/dt/1
  Delay1/1 -> Sum6/1
  "if we went through a \"step\""/1 -> Hold this value/Action
  Hold this value/1(Out1) -> divide by delta T/1
  Sum6/1 -> "if we went through a \"step\""/1, Hold this value/1(In1)
  y(t)/1 -> Sum6/2, Delay1/2, Delay1/1

== system Template_v4_00_2023a_Jetson/Phase #3: Experiment/Change RED Behavior/Sub-Phase #4/RED+ARM/Passthrough for Experiment ==
  q1_desired : Inport
  q2_desired : Inport  Port=2
  q3_desired : Inport  Port=3
  Action Port : ActionPort  ActionPortLabel=else
  q1_command : Outport
  q2_command : Outport  Port=2
  q3_command : Outport  Port=3
  wires:
  q3_desired/1 -> q3_command/1
  q1_desired/1 -> q1_command/1
  q2_desired/1 -> q2_command/1

== system Template_v4_00_2023a_Jetson/Phase #3: Experiment/Change RED Behavior/Sub-Phase #4/RED+ARM/Simulated Position Controller ==
  q1_desired : Inport
  q2_desired : Inport  Port=2
  q3_desired : Inport  Port=3
  Action Port : ActionPort  ActionPortLabel=if(u1 == 1)
  Custom Discrete PD (Elbow) : Subsystem
  Custom Discrete PD (Shoulder) : Subsystem
  Custom Discrete PD (Wrist) : Subsystem
  Data Store Read : DataStoreRead  DataStoreName=RED_Rz_Shoulder  IndexOptions=Index vector (dialog)  Indices=1  OutputSizes=1
  Data Store Read5 : DataStoreRead  DataStoreName=RED_Rz_Elbow  IndexOptions=Index vector (dialog)  Indices=1  OutputSizes=1
  Data Store Read6 : DataStoreRead  DataStoreName=RED_Rz_Wrist  IndexOptions=Index vector (dialog)  Indices=1  OutputSizes=1
  Saturation : Saturate  UpperLimit=Tz_lim_sharm  LowerLimit=-Tz_lim_sharm
  Saturation1 : Saturate  UpperLimit=Tz_lim_elarm  LowerLimit=-Tz_lim_elarm
  Saturation3 : Saturate  UpperLimit=Tz_lim_wrarm  LowerLimit=-Tz_lim_wrarm
  Subtract2 : Sum  Inputs=+-
  Subtract3 : Sum  Inputs=+-
  Subtract4 : Sum  Inputs=+-
  q1_command : Outport
  q2_command : Outport  Port=2
  q3_command : Outport  Port=3
  wires:
  Saturation3/1 -> q3_command/1
  Subtract4/1 -> Custom Discrete PD (Wrist)/1(ey)
  Custom Discrete PD (Shoulder)/1(Fx) -> Saturation/1
  Custom Discrete PD (Elbow)/1(Fy) -> Saturation1/1
  Saturation/1 -> q1_command/1
  Subtract2/1 -> Custom Discrete PD (Shoulder)/1(ex)
  Saturation1/1 -> q2_command/1
  Custom Discrete PD (Wrist)/1(Fy) -> Saturation3/1
  Subtract3/1 -> Custom Discrete PD (Elbow)/1(ey)
  Data Store Read/1 -> Subtract2/2
  Data Store Read5/1 -> Subtract3/2
  Data Store Read6/1 -> Subtract4/2
  q1_desired/1 -> Subtract2/1
  q2_desired/1 -> Subtract3/1
  q3_desired/1 -> Subtract4/1

== system Template_v4_00_2023a_Jetson/Phase #3: Experiment/Change RED Behavior/Sub-Phase #4/RED_Rz Desired/Subsystem ==
  Constant1 : Constant  Value=Phase2_End  SampleTime=-1
  Subtract : Sum  Inputs=+-
  Universal_Time : DataStoreRead  DataStoreName=Univ_Time  IndexOptions=Index vector (dialog)  Indices=1  OutputSizes=1
  Time : Outport  VectorParamsAs1DForOutWhenUnconnected=off
  wires:
  Universal_Time/1 -> Subtract/1
  Subtract/1 -> Time/1
  Constant1/1 -> Subtract/2

== system Template_v4_00_2023a_Jetson/Phase #3: Experiment/Change RED Behavior/Sub-Phase #4/RED_Rz Desired/Wrap ==
  unwrapped : Inport
  MATLAB Function : MATLAB Function  TreatAsAtomicUnit=on
  wrapped : Outport  VectorParamsAs1DForOutWhenUnconnected=off
  wires:
  MATLAB Function/1(wrappedAngle) -> wrapped/1
  unwrapped/1 -> MATLAB Function/1(u)

== system Template_v4_00_2023a_Jetson/Phase #3: Experiment/Change RED Behavior/Sub-Phase #4/Subsystem1/Subsystem ==
  Universal_Time : DataStoreRead  DataStoreName=Univ_Time  IndexOptions=Index vector (dialog)  Indices=1  OutputSizes=1
  Time : Outport  VectorParamsAs1DForOutWhenUnconnected=off
  wires:
  Universal_Time/1 -> Time/1

== system Template_v4_00_2023a_Jetson/Phase #4: Return Home/Change BLACK Behavior/Custom Discrete PD (Attitude)/x_dot -> x1/Hold this value ==
  In1 : Inport
  Action Port : ActionPort  ActionPortLabel=if(u1 ~= 0)
  Out1 : Outport  VectorParamsAs1DForOutWhenUnconnected=off
  wires:
  In1/1 -> Out1/1

== system Template_v4_00_2023a_Jetson/Phase #4: Return Home/Change BLACK Behavior/Custom Discrete PD (X-Position)/x_dot -> x1/Hold this value ==
  In1 : Inport
  Action Port : ActionPort  ActionPortLabel=if(u1 ~= 0)
  Out1 : Outport  VectorParamsAs1DForOutWhenUnconnected=off
  wires:
  In1/1 -> Out1/1

== system Template_v4_00_2023a_Jetson/Phase #4: Return Home/Change BLACK Behavior/Custom Discrete PD (Y-Position)/x_dot -> x1/Hold this value ==
  In1 : Inport
  Action Port : ActionPort  ActionPortLabel=if(u1 ~= 0)
  Out1 : Outport  VectorParamsAs1DForOutWhenUnconnected=off
  wires:
  In1/1 -> Out1/1

== system Template_v4_00_2023a_Jetson/Phase #4: Return Home/Change BLUE Behavior/Custom Discrete PD (Attitude)/x_dot -> x1/Hold this value ==
  In1 : Inport
  Action Port : ActionPort  ActionPortLabel=if(u1 ~= 0)
  Out1 : Outport  VectorParamsAs1DForOutWhenUnconnected=off
  wires:
  In1/1 -> Out1/1

== system Template_v4_00_2023a_Jetson/Phase #4: Return Home/Change BLUE Behavior/Custom Discrete PD (X-Position)/x_dot -> x1/Hold this value ==
  In1 : Inport
  Action Port : ActionPort  ActionPortLabel=if(u1 ~= 0)
  Out1 : Outport  VectorParamsAs1DForOutWhenUnconnected=off
  wires:
  In1/1 -> Out1/1

== system Template_v4_00_2023a_Jetson/Phase #4: Return Home/Change BLUE Behavior/Custom Discrete PD (Y-Position)/x_dot -> x1/Hold this value ==
  In1 : Inport
  Action Port : ActionPort  ActionPortLabel=if(u1 ~= 0)
  Out1 : Outport  VectorParamsAs1DForOutWhenUnconnected=off
  wires:
  In1/1 -> Out1/1

== system Template_v4_00_2023a_Jetson/Phase #4: Return Home/Change RED Behavior/Custom Discrete PD (Attitude)/x_dot -> x2/Hold this value ==
  In1 : Inport
  Action Port : ActionPort  ActionPortLabel=if(u1 ~= 0)
  Out1 : Outport  VectorParamsAs1DForOutWhenUnconnected=off
  wires:
  In1/1 -> Out1/1

== system Template_v4_00_2023a_Jetson/Phase #4: Return Home/Change RED Behavior/Custom Discrete PD (X-Position)/x_dot -> x2/Hold this value ==
  In1 : Inport
  Action Port : ActionPort  ActionPortLabel=if(u1 ~= 0)
  Out1 : Outport  VectorParamsAs1DForOutWhenUnconnected=off
  wires:
  In1/1 -> Out1/1

== system Template_v4_00_2023a_Jetson/Phase #4: Return Home/Change RED Behavior/Custom Discrete PD (Y-Position)/x_dot -> x2/Hold this value ==
  In1 : Inport
  Action Port : ActionPort  ActionPortLabel=if(u1 ~= 0)
  Out1 : Outport  VectorParamsAs1DForOutWhenUnconnected=off
  wires:
  In1/1 -> Out1/1

== system Template_v4_00_2023a_Jetson/Phase #4: Return Home/Change RED Behavior/RED+ARM/Simulated Position Controller/Custom Discrete PD (Elbow) ==
  ey : Inport
  Sum3 : Sum
  kd_elarm : Gain  Gain=Kd_elarm
  kp_elarm : Gain  Gain=Kp_elarm
  "x_dot -> x2" : Subsystem
  Fy : Outport  VectorParamsAs1DForOutWhenUnconnected=off
  wires:
  kd_elarm/1 -> Sum3/1
  Sum3/1 -> Fy/1
  kp_elarm/1 -> Sum3/2
  "x_dot -> x2"/1(dy(t)/dt) -> kd_elarm/1
  ey/1 -> "x_dot -> x2"/1(y(t)), kp_elarm/1

== system Template_v4_00_2023a_Jetson/Phase #4: Return Home/Change RED Behavior/RED+ARM/Simulated Position Controller/Custom Discrete PD (Shoulder) ==
  ex : Inport
  Sum3 : Sum
  kd_sharm : Gain  Gain=Kd_sharm
  kp_sharm : Gain  Gain=Kp_sharm
  "x_dot -> x2" : Subsystem
  Fx : Outport  VectorParamsAs1DForOutWhenUnconnected=off
  wires:
  kd_sharm/1 -> Sum3/1
  ex/1 -> "x_dot -> x2"/1(y(t)), kp_sharm/1
  kp_sharm/1 -> Sum3/2
  "x_dot -> x2"/1(dy(t)/dt) -> kd_sharm/1
  Sum3/1 -> Fx/1

== system Template_v4_00_2023a_Jetson/Phase #4: Return Home/Change RED Behavior/RED+ARM/Simulated Position Controller/Custom Discrete PD (Wrist) ==
  ey : Inport
  Sum3 : Sum
  kd_wrarm : Gain  Gain=Kd_wrarm
  kp_wrarm : Gain  Gain=Kp_wrarm
  "x_dot -> x2" : Subsystem
  Fy : Outport  VectorParamsAs1DForOutWhenUnconnected=off
  wires:
  kd_wrarm/1 -> Sum3/1
  Sum3/1 -> Fy/1
  kp_wrarm/1 -> Sum3/2
  "x_dot -> x2"/1(dy(t)/dt) -> kd_wrarm/1
  ey/1 -> "x_dot -> x2"/1(y(t)), kp_wrarm/1

== system Template_v4_00_2023a_Jetson/Phase #5: Hold Home/Change BLACK Behavior/Custom Discrete PD (Attitude)/x_dot -> x1/Hold this value ==
  In1 : Inport
  Action Port : ActionPort  ActionPortLabel=if(u1 ~= 0)
  Out1 : Outport  VectorParamsAs1DForOutWhenUnconnected=off
  wires:
  In1/1 -> Out1/1

== system Template_v4_00_2023a_Jetson/Phase #5: Hold Home/Change BLACK Behavior/Custom Discrete PD (X-Position)/x_dot -> x1/Hold this value ==
  In1 : Inport
  Action Port : ActionPort  ActionPortLabel=if(u1 ~= 0)
  Out1 : Outport  VectorParamsAs1DForOutWhenUnconnected=off
  wires:
  In1/1 -> Out1/1

== system Template_v4_00_2023a_Jetson/Phase #5: Hold Home/Change BLACK Behavior/Custom Discrete PD (Y-Position)/x_dot -> x1/Hold this value ==
  In1 : Inport
  Action Port : ActionPort  ActionPortLabel=if(u1 ~= 0)
  Out1 : Outport  VectorParamsAs1DForOutWhenUnconnected=off
  wires:
  In1/1 -> Out1/1

== system Template_v4_00_2023a_Jetson/Phase #5: Hold Home/Change BLUE Behavior/Custom Discrete PD (Attitude)/x_dot -> x1/Hold this value ==
  In1 : Inport
  Action Port : ActionPort  ActionPortLabel=if(u1 ~= 0)
  Out1 : Outport  VectorParamsAs1DForOutWhenUnconnected=off
  wires:
  In1/1 -> Out1/1
